simulink model "Simulink_Modell"  (R2020b)
settings: Solver=VariableStepAuto  StartTime=0.0  StopTime=1  MaxStep=0.000125  RelTol=1e-4  AbsTol=0.0000001
libraries: pid_lib x2
settings Model: Creator=Mei  LastModifiedBy=16007

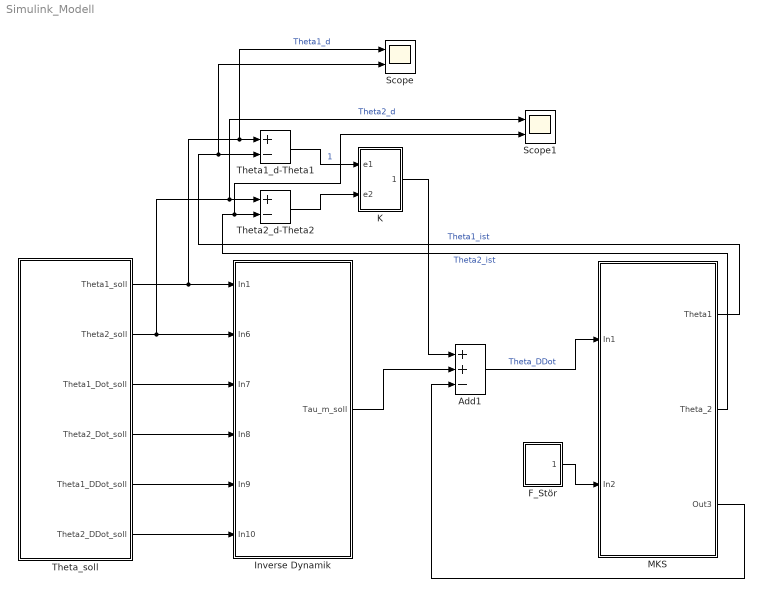
== system Simulink_Modell ==
  Add1 : Sum  Inputs=++-
  F_Stör : Subsystem
  Inverse Dynamik : Subsystem
  K : Subsystem
  MKS : Subsystem
  Scope : Scope  NumInputPorts=2
  Scope1 : Scope  NumInputPorts=2
  Theta1_d-Theta1 : Sum  Inputs=+-
  Theta2_d-Theta2 : Sum  Inputs=+-
  Theta_soll : Subsystem
  wires:
  Theta_soll/1(Theta1_soll) -> Scope/1, Theta1_d-Theta1/1, Inverse Dynamik/1(In1)  "Theta1_d"
  Theta_soll/2(Theta2_soll) -> Scope1/1, Theta2_d-Theta2/1, Inverse Dynamik/2(In6)  "Theta2_d"
  Theta_soll/3(Theta1_Dot_soll) -> Inverse Dynamik/3(In7)
  Theta_soll/4(Theta2_Dot_soll) -> Inverse Dynamik/4(In8)
  Theta_soll/5(Theta1_DDot_soll) -> Inverse Dynamik/5(In9)
  Theta_soll/6(Theta2_DDot_soll) -> Inverse Dynamik/6(In10)
  Add1/1 -> MKS/1(In1)  "Theta_DDot"
  F_Stör/1(1) -> MKS/2(In2)
  MKS/1(Theta1) -> Scope/2, Theta1_d-Theta1/2  "Theta1_ist"
  MKS/2(Theta_2) -> Scope1/2, Theta2_d-Theta2/2  "Theta2_ist"
  Theta1_d-Theta1/1 -> K/1(e1)  "1"
  Theta2_d-Theta2/1 -> K/2(e2)
  K/1(Out1) -> Add1/1
  Inverse Dynamik/1(Tau_m_soll) -> Add1/2
  MKS/3(Out3) -> Add1/3

== system Simulink_Modell/F_Stör ==
  Constant8 : Constant
  MATLAB Function : MATLAB Function  TreatAsAtomicUnit=on
  1 : Outport
  wires:
  Constant8/1 -> MATLAB Function/1(u)
  MATLAB Function/1(Fstoer) -> 1/1

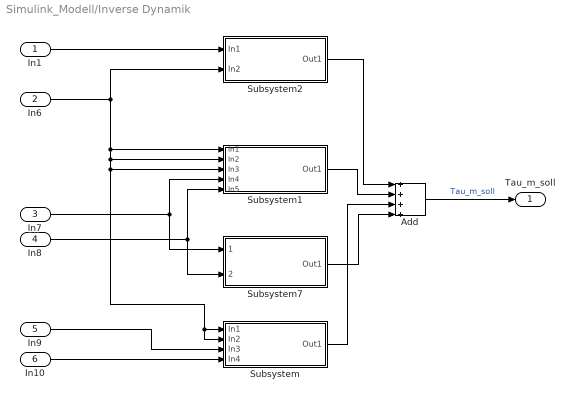
== system Simulink_Modell/Inverse Dynamik ==
  In1 : Inport
  In6 : Inport  Port=2
  In7 : Inport  Port=3
  In8 : Inport  Port=4
  In9 : Inport  Port=5
  In10 : Inport  Port=6
  Add : Sum  Inputs=++++
  Subsystem : Subsystem
  Subsystem1 : Subsystem
  Subsystem2 : Subsystem
  Subsystem7 : Subsystem
  Tau_m_soll : Outport
  wires:
  In7/1 -> Subsystem1/4(In4), Subsystem7/1(1)
  In8/1 -> Subsystem1/5(In5), Subsystem7/2(2)
  Add/1 -> Tau_m_soll/1  "Tau_m_soll"
  Subsystem/1(Out1) -> Add/3
  Subsystem1/1(Out1) -> Add/2
  Subsystem2/1(Out1) -> Add/1
  In6/1 -> Subsystem/2(In2), Subsystem/1(In1), Subsystem1/3(In3), Subsystem1/2(In2), Subsystem1/1(In1), Subsystem2/2(In2)
  Subsystem7/1(Out1) -> Add/4
  In1/1 -> Subsystem2/1(In1)
  In10/1 -> Subsystem/4(In4)
  In9/1 -> Subsystem/3(In3)

== system Simulink_Modell/K ==
  e1 : Inport
  e2 : Inport  Port=2
  Mux : Mux  Inputs=2
  PID1 : pid_lib/PID Controller  Controller=PID  Form=Parallel  TimeDomain=Discrete-time  UseExternalTs=off  SampleTime=-1  IntegratorMethod=Forward Euler  FilterMethod=Forward Euler  ControllerParametersSource=internal  P=300  I=10  D=10  UseFilter=on  N=100  TunerSelectOption=Transfer Function Based (PID Tuner App)  InitialConditionSource=internal  InitialConditionForIntegrator=0  InitialConditionForFilter=0  DifferentiatorICPrevScaledInput=0  ExternalReset=none  TrackingMode=off  Kt=1  LimitOutput=off  SatLimitsSource=internal  UpperSaturationLimit=inf  LowerSaturationLimit=-inf  LinearizeAsGain=on  AntiWindupMode=none  Kb=1  POutMin=[]  POutMax=[]  IOutMin=[]  IOutMax=[]  DOutMin=[]  DOutMax=[]  NOutMin=[]  NOutMax=[]  SumOutMin=[]  SumOutMax=[]  SaturationOutMin=[]  SaturationOutMax=[]  PParamMin=[]  PParamMax=[]  IParamMin=[]  IParamMax=[]  DParamMin=[]  DParamMax=[]  NParamMin=[]  NParamMax=[]  KbParamMin=[]  KbParamMax=[]  KtParamMin=[]  KtParamMax=[]  KbOutMin=[]  KbOutMax=[]  KtOutMin=[]  KtOutMax=[]  IntegratorOutMin=[]  IntegratorOutMax=[]  FilterOutMin=[]  FilterOutMax=[]  SumI1OutMin=[]  SumI1OutMax=[]  SumI2OutMin=[]  SumI2OutMax=[]  SumI3OutMin=[]  SumI3OutMax=[]  SumI4OutMin=[]  SumI4OutMax=[]  SumDOutMin=[]  SumDOutMax=[]  DifferentiatorOutMin=[]  DifferentiatorOutMax=[]  FilterDiffOutCoefMin=[]  FilterDiffOutCoefMax=[]  ReciprocalOutMin=[]  ReciprocalOutMax=[]  SumDenOutMin=[]  SumDenOutMax=[]  SumNumOutMin=[]  SumNumOutMax=[]  DivideOutMin=[]  DivideOutMax=[]  UdiffTsProdOutMin=[]  UdiffTsProdOutMax=[]  NTsProdOutMin=[]  NTsProdOutMax=[]  UintegralTsProdOutMin=[]  UintegralTsProdOutMax=[]  UngainTsProdOutMin=[]  UngainTsProdOutMax=[]  IntegratorContinuousStateAttributes=''  IntegratorStateMustResolveToSignalObject=off  IntegratorRTWStateStorageClass=Auto  FilterContinuousStateAttributes=''  FilterStateMustResolveToSignalObject=off  FilterRTWStateStorageClass=Auto  ParallelPVariant=InternalParameters  IdealPVariant=Disabled  IVariant=InternalParameters  DVariant=InternalParameters  IntegratorVariant=Discrete  SatVariant=Disabled  AWVariant=Passthrough  PCopyVariant=Disabled  TRVariant=Disabled  FdbkBlocksVariant=Forward  IdealPFdbkVariant=Disabled  SatFdbkVariant=Disabled  DerivativeFilterVariant=ForwardEulerFilter  NVariant=InternalParameters  NCopyVariant=Disabled  FilterICVariant=InternalICsFilter  IntegratorICVariant=InternalICs  ExternalResetVariant=Disabled  TRSumVariant=Passthrough  SumFdbkVariant=Disabled  SumVariant=Sum_PID  TsampFilterVariant=InternalTs  TsampNgainVariant=Passthrough  TsampIntegralVariant=Passthrough  ExternalSaturationOutDataTypeStr=Inherit: Same as second input
  PID2 : pid_lib/PID Controller  Controller=PID  Form=Parallel  TimeDomain=Discrete-time  UseExternalTs=off  SampleTime=-1  IntegratorMethod=Forward Euler  FilterMethod=Forward Euler  ControllerParametersSource=internal  P=1500  I=100  D=10  UseFilter=on  N=100  TunerSelectOption=Transfer Function Based (PID Tuner App)  InitialConditionSource=internal  InitialConditionForIntegrator=0  InitialConditionForFilter=0  DifferentiatorICPrevScaledInput=0  ExternalReset=none  TrackingMode=off  Kt=1  LimitOutput=off  SatLimitsSource=internal  UpperSaturationLimit=inf  LowerSaturationLimit=-inf  LinearizeAsGain=on  AntiWindupMode=none  Kb=1  POutMin=[]  POutMax=[]  IOutMin=[]  IOutMax=[]  DOutMin=[]  DOutMax=[]  NOutMin=[]  NOutMax=[]  SumOutMin=[]  SumOutMax=[]  SaturationOutMin=[]  SaturationOutMax=[]  PParamMin=[]  PParamMax=[]  IParamMin=[]  IParamMax=[]  DParamMin=[]  DParamMax=[]  NParamMin=[]  NParamMax=[]  KbParamMin=[]  KbParamMax=[]  KtParamMin=[]  KtParamMax=[]  KbOutMin=[]  KbOutMax=[]  KtOutMin=[]  KtOutMax=[]  IntegratorOutMin=[]  IntegratorOutMax=[]  FilterOutMin=[]  FilterOutMax=[]  SumI1OutMin=[]  SumI1OutMax=[]  SumI2OutMin=[]  SumI2OutMax=[]  SumI3OutMin=[]  SumI3OutMax=[]  SumI4OutMin=[]  SumI4OutMax=[]  SumDOutMin=[]  SumDOutMax=[]  DifferentiatorOutMin=[]  DifferentiatorOutMax=[]  FilterDiffOutCoefMin=[]  FilterDiffOutCoefMax=[]  ReciprocalOutMin=[]  ReciprocalOutMax=[]  SumDenOutMin=[]  SumDenOutMax=[]  SumNumOutMin=[]  SumNumOutMax=[]  DivideOutMin=[]  DivideOutMax=[]  UdiffTsProdOutMin=[]  UdiffTsProdOutMax=[]  NTsProdOutMin=[]  NTsProdOutMax=[]  UintegralTsProdOutMin=[]  UintegralTsProdOutMax=[]  UngainTsProdOutMin=[]  UngainTsProdOutMax=[]  IntegratorContinuousStateAttributes=''  IntegratorStateMustResolveToSignalObject=off  IntegratorRTWStateStorageClass=Auto  FilterContinuousStateAttributes=''  FilterStateMustResolveToSignalObject=off  FilterRTWStateStorageClass=Auto  ParallelPVariant=InternalParameters  IdealPVariant=Disabled  IVariant=InternalParameters  DVariant=InternalParameters  IntegratorVariant=Discrete  SatVariant=Disabled  AWVariant=Passthrough  PCopyVariant=Disabled  TRVariant=Disabled  FdbkBlocksVariant=Forward  IdealPFdbkVariant=Disabled  SatFdbkVariant=Disabled  DerivativeFilterVariant=ForwardEulerFilter  NVariant=InternalParameters  NCopyVariant=Disabled  FilterICVariant=InternalICsFilter  IntegratorICVariant=InternalICs  ExternalResetVariant=Disabled  TRSumVariant=Passthrough  SumFdbkVariant=Disabled  SumVariant=Sum_PID  TsampFilterVariant=InternalTs  TsampNgainVariant=Passthrough  TsampIntegralVariant=Passthrough  ExternalSaturationOutDataTypeStr=Inherit: Same as second input
  Out1 : Outport
  wires:
  PID1/1 -> Mux/1
  e1/1 -> PID1/1
  PID2/1 -> Mux/2
  e2/1 -> PID2/1
  Mux/1 -> Out1/1

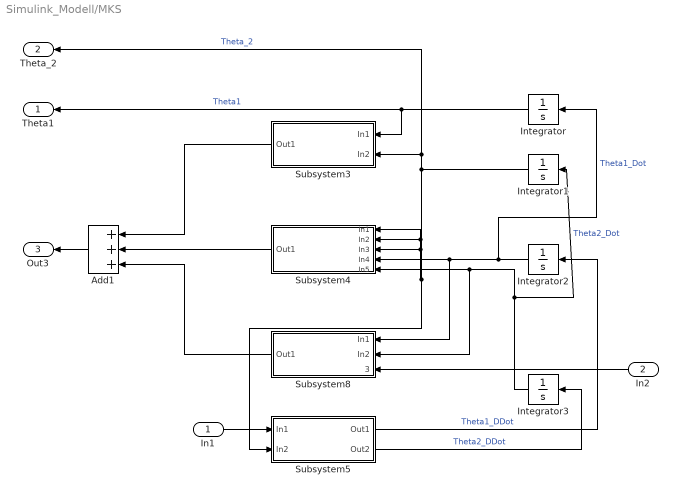
== system Simulink_Modell/MKS ==
  In1 : Inport
  In2 : Inport  Port=2
  Add1 : Sum  Inputs=+++
  Integrator{,1..3} (4 alike) : Integrator
  Subsystem3 : Subsystem
  Subsystem4 : Subsystem
  Subsystem5 : Subsystem
  Subsystem8 : Subsystem
  Theta1 : Outport
  Theta_2 : Outport  Port=2
  Out3 : Outport  Port=3
  wires:
  Integrator3/1 -> Integrator1/1, Subsystem4/5(In5), Subsystem8/2(In2)  "Theta2_Dot"
  Subsystem4/1(Out1) -> Add1/2
  Integrator2/1 -> Subsystem8/1(In1), Subsystem4/4(In4), Integrator/1  "Theta1_Dot"
  Subsystem5/2(Out2) -> Integrator3/1  "Theta2_DDot"
  Integrator1/1 -> Subsystem4/1(In1), Subsystem4/2(In2), Subsystem4/3(In3), Subsystem5/2(In2), Theta_2/1, Subsystem3/2(In2)  "Theta_2"
  Integrator/1 -> Theta1/1, Subsystem3/1(In1)  "Theta1"
  Subsystem5/1(Out1) -> Integrator2/1  "Theta1_DDot"
  In1/1 -> Subsystem5/1(In1)
  Subsystem3/1(Out1) -> Add1/1
  Subsystem8/1(Out1) -> Add1/3
  In2/1 -> Subsystem8/3(3)
  Add1/1 -> Out3/1

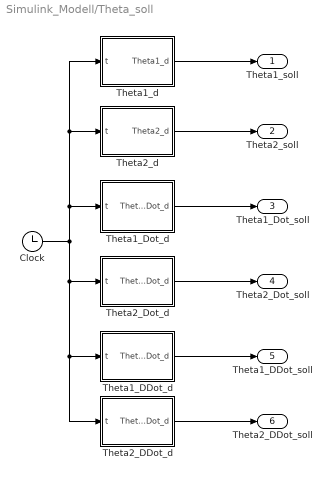
== system Simulink_Modell/Theta_soll ==
  Clock : Clock
  Theta1_DDot_d : MATLAB Function  TreatAsAtomicUnit=on
  Theta1_Dot_d : MATLAB Function  TreatAsAtomicUnit=on
  Theta1_d : MATLAB Function  TreatAsAtomicUnit=on
  Theta2_DDot_d : MATLAB Function  TreatAsAtomicUnit=on
  Theta2_Dot_d : MATLAB Function  TreatAsAtomicUnit=on
  Theta2_d : MATLAB Function  TreatAsAtomicUnit=on
  Theta1_soll : Outport
  Theta2_soll : Outport  Port=2
  Theta1_Dot_soll : Outport  Port=3
  Theta2_Dot_soll : Outport  Port=4
  Theta1_DDot_soll : Outport  Port=5
  Theta2_DDot_soll : Outport  Port=6
  wires:
  Theta1_Dot_d/1(Theta1_Dot_d) -> Theta1_Dot_soll/1
  Clock/1 -> Theta1_d/1(t), Theta2_d/1(t), Theta1_Dot_d/1(t), Theta2_DDot_d/1(t), Theta1_DDot_d/1(t), Theta2_Dot_d/1(t)
  Theta1_DDot_d/1(Theta1_DDot_d) -> Theta1_DDot_soll/1
  Theta1_d/1(Theta1_d) -> Theta1_soll/1
  Theta2_DDot_d/1(Theta2_DDot_d) -> Theta2_DDot_soll/1
  Theta2_Dot_d/1(Theta2_Dot_d) -> Theta2_Dot_soll/1
  Theta2_d/1(Theta2_d) -> Theta2_soll/1

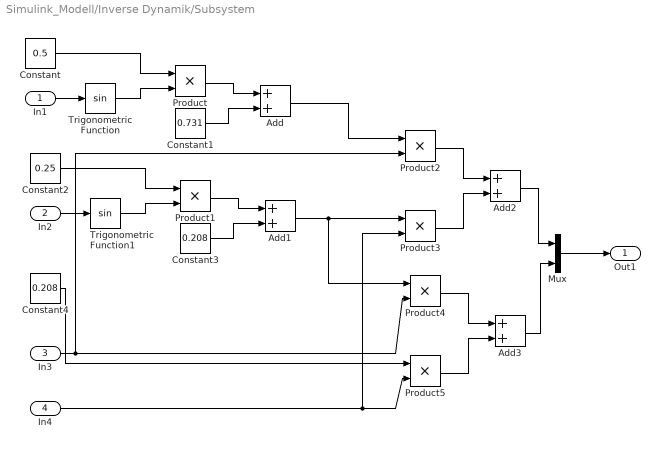
== system Simulink_Modell/Inverse Dynamik/Subsystem ==
  In1 : Inport
  In2 : Inport  Port=2
  In3 : Inport  Port=3
  In4 : Inport  Port=4
  Add{,1..3} (4 alike) : Sum
  Constant : Constant  Value=0.5
  Constant1 : Constant  Value=0.731
  Constant2 : Constant  Value=0.25
  Constant3 : Constant  Value=0.208
  Constant4 : Constant  Value=0.208
  Mux : Mux  Inputs=2
  Product{,1..5} (6 alike) : Product
  Trigonometric Function : Trigonometry
  Trigonometric Function1 : Trigonometry
  Out1 : Outport
  wires:
  Constant/1 -> Product/1
  Product/1 -> Add/1
  Constant1/1 -> Add/2
  In1/1 -> Trigonometric Function/1
  Trigonometric Function/1 -> Product/2
  Product1/1 -> Add1/1
  Constant3/1 -> Add1/2
  Constant2/1 -> Product1/1
  Trigonometric Function1/1 -> Product1/2
  In2/1 -> Trigonometric Function1/1
  In3/1 -> Product2/2, Product4/2
  Add/1 -> Product2/1
  Add1/1 -> Product4/1, Product3/1
  In4/1 -> Product3/2, Product5/2
  Product2/1 -> Add2/1
  Product3/1 -> Add2/2
  Product4/1 -> Add3/1
  Product5/1 -> Add3/2
  Constant4/1 -> Product5/1
  Add2/1 -> Mux/1
  Add3/1 -> Mux/2
  Mux/1 -> Out1/1

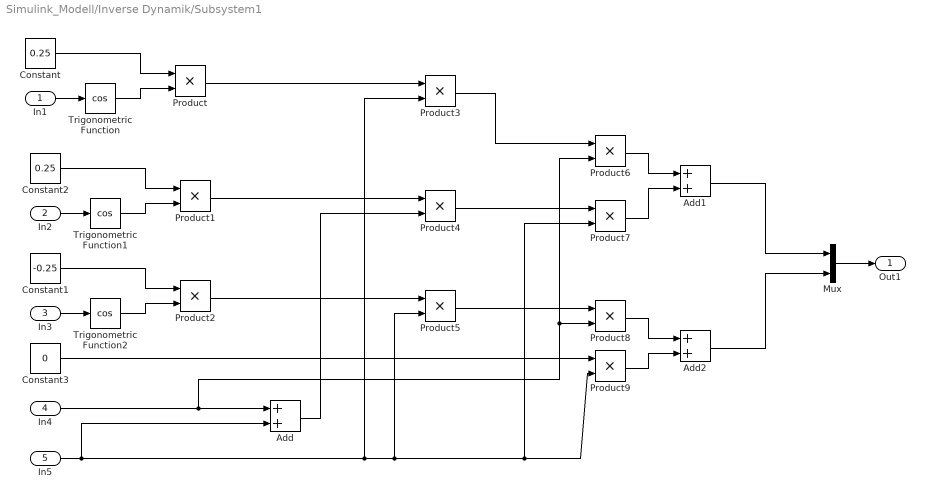
== system Simulink_Modell/Inverse Dynamik/Subsystem1 ==
  In1 : Inport
  In2 : Inport  Port=2
  In3 : Inport  Port=3
  In4 : Inport  Port=4
  In5 : Inport  Port=5
  Add : Sum
  Add1 : Sum
  Add2 : Sum
  Constant : Constant  Value=0.25
  Constant1 : Constant  Value=-0.25
  Constant2 : Constant  Value=0.25
  Constant3 : Constant  Value=0
  Mux : Mux  Inputs=2
  Product{,1..9} (10 alike) : Product
  Trigonometric Function : Trigonometry  Operator=cos
  Trigonometric Function1 : Trigonometry  Operator=cos
  Trigonometric Function2 : Trigonometry  Operator=cos
  Out1 : Outport
  wires:
  Constant/1 -> Product/1
  Trigonometric Function1/1 -> Product1/2
  Constant2/1 -> Product1/1
  In2/1 -> Trigonometric Function1/1
  Trigonometric Function/1 -> Product/2
  In1/1 -> Trigonometric Function/1
  In3/1 -> Trigonometric Function2/1
  Trigonometric Function2/1 -> Product2/2
  Constant1/1 -> Product2/1
  Product/1 -> Product3/1
  In5/1 -> Add/2, Product5/2, Product9/2, Product7/2, Product3/2
  Product1/1 -> Product4/1
  In4/1 -> Product6/2, Product8/2, Add/1
  Add/1 -> Product4/2
  Product2/1 -> Product5/1
  Product3/1 -> Product6/1
  Product4/1 -> Product7/1
  Product7/1 -> Add1/2
  Product6/1 -> Add1/1
  Product9/1 -> Add2/2
  Product8/1 -> Add2/1
  Product5/1 -> Product8/1
  Constant3/1 -> Product9/1
  Add2/1 -> Mux/2
  Add1/1 -> Mux/1
  Mux/1 -> Out1/1

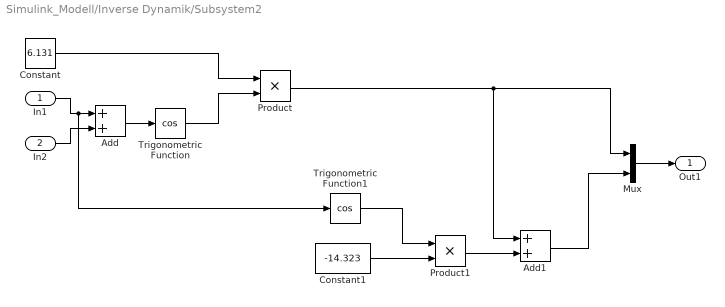
== system Simulink_Modell/Inverse Dynamik/Subsystem2 ==
  In1 : Inport
  In2 : Inport  Port=2
  Add : Sum
  Add1 : Sum
  Constant : Constant  Value=6.131
  Constant1 : Constant  Value=-14.323
  Mux : Mux  Inputs=2
  Product : Product
  Product1 : Product
  Trigonometric Function : Trigonometry  Operator=cos
  Trigonometric Function1 : Trigonometry  Operator=cos
  Out1 : Outport
  wires:
  Trigonometric Function/1 -> Product/2
  Constant/1 -> Product/1
  In1/1 -> Trigonometric Function1/1, Add/1
  In2/1 -> Add/2
  Add/1 -> Trigonometric Function/1
  Trigonometric Function1/1 -> Product1/1
  Constant1/1 -> Product1/2
  Product1/1 -> Add1/2
  Product/1 -> Mux/1, Add1/1
  Add1/1 -> Mux/2
  Mux/1 -> Out1/1

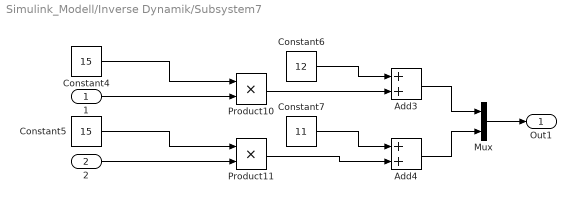
== system Simulink_Modell/Inverse Dynamik/Subsystem7 ==
  1 : Inport
  2 : Inport  Port=2
  Add3 : Sum
  Add4 : Sum
  Constant4 : Constant  Value=15
  Constant5 : Constant  Value=15
  Constant6 : Constant  Value=12
  Constant7 : Constant  Value=11
  Mux : Mux  Inputs=2
  Product10 : Product
  Product11 : Product
  Out1 : Outport
  wires:
  Constant6/1 -> Add3/1
  Product10/1 -> Add3/2
  Add3/1 -> Mux/1
  Constant7/1 -> Add4/1
  Product11/1 -> Add4/2
  Constant4/1 -> Product10/1
  2/1 -> Product11/2
  Constant5/1 -> Product11/1
  1/1 -> Product10/2
  Add4/1 -> Mux/2
  Mux/1 -> Out1/1

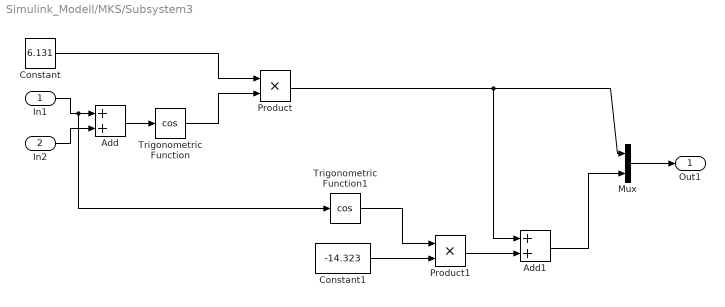
== system Simulink_Modell/MKS/Subsystem3 ==
  In1 : Inport
  In2 : Inport  Port=2
  Add : Sum
  Add1 : Sum
  Constant : Constant  Value=6.131
  Constant1 : Constant  Value=-14.323
  Mux : Mux  Inputs=2
  Product : Product
  Product1 : Product
  Trigonometric Function : Trigonometry  Operator=cos
  Trigonometric Function1 : Trigonometry  Operator=cos
  Out1 : Outport
  wires:
  Trigonometric Function/1 -> Product/2
  Constant/1 -> Product/1
  In1/1 -> Trigonometric Function1/1, Add/1
  In2/1 -> Add/2
  Add/1 -> Trigonometric Function/1
  Trigonometric Function1/1 -> Product1/1
  Constant1/1 -> Product1/2
  Product1/1 -> Add1/2
  Product/1 -> Mux/1, Add1/1
  Add1/1 -> Mux/2
  Mux/1 -> Out1/1

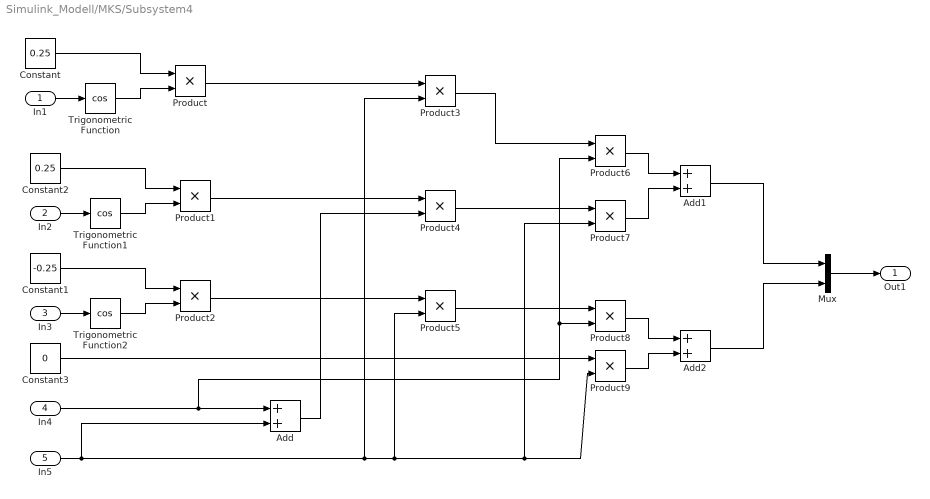
== system Simulink_Modell/MKS/Subsystem4 ==
  In1 : Inport
  In2 : Inport  Port=2
  In3 : Inport  Port=3
  In4 : Inport  Port=4
  In5 : Inport  Port=5
  Add : Sum
  Add1 : Sum
  Add2 : Sum
  Constant : Constant  Value=0.25
  Constant1 : Constant  Value=-0.25
  Constant2 : Constant  Value=0.25
  Constant3 : Constant  Value=0
  Mux : Mux  Inputs=2
  Product{,1..9} (10 alike) : Product
  Trigonometric Function : Trigonometry  Operator=cos
  Trigonometric Function1 : Trigonometry  Operator=cos
  Trigonometric Function2 : Trigonometry  Operator=cos
  Out1 : Outport
  wires:
  Constant/1 -> Product/1
  Trigonometric Function1/1 -> Product1/2
  Constant2/1 -> Product1/1
  In2/1 -> Trigonometric Function1/1
  Trigonometric Function/1 -> Product/2
  In1/1 -> Trigonometric Function/1
  In3/1 -> Trigonometric Function2/1
  Trigonometric Function2/1 -> Product2/2
  Constant1/1 -> Product2/1
  Product/1 -> Product3/1
  In5/1 -> Add/2, Product5/2, Product9/2, Product7/2, Product3/2
  Product1/1 -> Product4/1
  In4/1 -> Product6/2, Product8/2, Add/1
  Add/1 -> Product4/2
  Product2/1 -> Product5/1
  Product3/1 -> Product6/1
  Product4/1 -> Product7/1
  Product7/1 -> Add1/2
  Product6/1 -> Add1/1
  Product9/1 -> Add2/2
  Product8/1 -> Add2/1
  Product5/1 -> Product8/1
  Constant3/1 -> Product9/1
  Add2/1 -> Mux/2
  Add1/1 -> Mux/1
  Mux/1 -> Out1/1

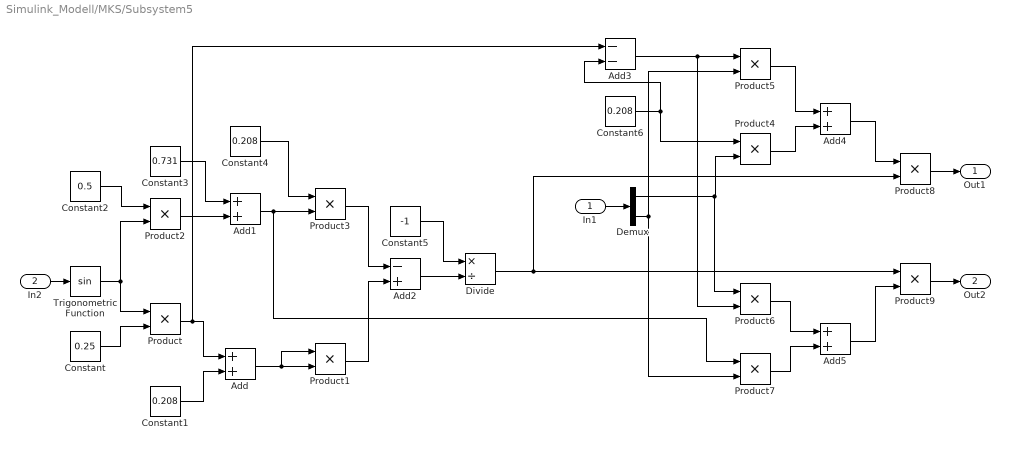
== system Simulink_Modell/MKS/Subsystem5 ==
  In1 : Inport
  In2 : Inport  Port=2
  Add{,1,4..5} (4 alike) : Sum
  Add2 : Sum  Inputs=-+
  Add3 : Sum  Inputs=--
  Constant : Constant  Value=0.25
  Constant1 : Constant  Value=0.208
  Constant2 : Constant  Value=0.5
  Constant3 : Constant  Value=0.731
  Constant4 : Constant  Value=0.208
  Constant5 : Constant  Value=-1
  Constant6 : Constant  Value=0.208
  Demux : Demux  Outputs=2
  Divide : Product  Inputs=*/
  Product{,1..9} (10 alike) : Product
  Trigonometric Function : Trigonometry
  Out1 : Outport
  Out2 : Outport  Port=2
  wires:
  In1/1 -> Demux/1
  In2/1 -> Trigonometric Function/1
  Trigonometric Function/1 -> Product2/2, Product/1
  Constant/1 -> Product/2
  Constant1/1 -> Add/2
  Product/1 -> Add3/1, Add/1
  Add/1 -> Product1/1, Product1/2
  Constant2/1 -> Product2/1
  Product2/1 -> Add1/2
  Constant3/1 -> Add1/1
  Add1/1 -> Product7/1, Product3/2
  Constant4/1 -> Product3/1
  Product1/1 -> Add2/2
  Product3/1 -> Add2/1
  Add2/1 -> Divide/2
  Constant5/1 -> Divide/1
  Constant6/1 -> Add3/2, Product4/1
  Demux/1 -> Product6/1, Product4/2
  Add3/1 -> Product5/1, Product6/2
  Demux/2 -> Product7/2, Product5/2
  Product5/1 -> Add4/1
  Product4/1 -> Add4/2
  Product6/1 -> Add5/1
  Product7/1 -> Add5/2
  Divide/1 -> Product9/1, Product8/2
  Add4/1 -> Product8/1
  Product8/1 -> Out1/1
  Add5/1 -> Product9/2
  Product9/1 -> Out2/1

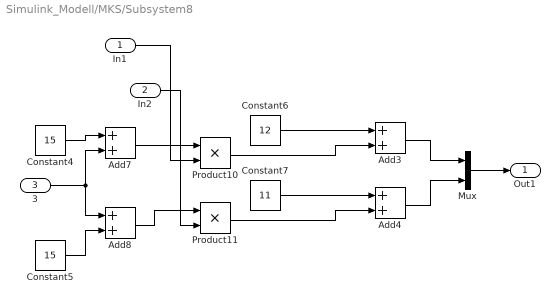
== system Simulink_Modell/MKS/Subsystem8 ==
  In1 : Inport
  In2 : Inport  Port=2
  3 : Inport  Port=3
  Add{3..4,7..8} (4 alike) : Sum
  Constant4 : Constant  Value=15
  Constant5 : Constant  Value=15
  Constant6 : Constant  Value=12
  Constant7 : Constant  Value=11
  Mux : Mux  Inputs=2
  Product10 : Product
  Product11 : Product
  Out1 : Outport
  wires:
  Constant5/1 -> Add8/2
  3/1 -> Add8/1, Add7/2
  Add8/1 -> Product11/1
  Product10/1 -> Add3/2
  Constant7/1 -> Add4/1
  Constant6/1 -> Add3/1
  Product11/1 -> Add4/2
  Constant4/1 -> Add7/1
  Add7/1 -> Product10/1
  Add4/1 -> Mux/2
  In2/1 -> Product11/2
  In1/1 -> Product10/2
  Add3/1 -> Mux/1
  Mux/1 -> Out1/1

== matlab function Simulink_Modell/Theta_soll/Theta1_d ==
  data: t input; Theta1_d output
function Theta1_d = fcn(t)
Theta1_d = -43.5*t.^2+29*t.^3;

== matlab function Simulink_Modell/Theta_soll/Theta1_Dot_d ==
  data: t input; Theta1_Dot_d output
function Theta1_Dot_d = fcn(t)
Theta1_Dot_d = -87*t+87*t^2;

== matlab function Simulink_Modell/Theta_soll/Theta2_Dot_d ==
  data: t input; Theta2_Dot_d output
function Theta2_Dot_d = fcn(t)
Theta2_Dot_d = 96*t-96*t^2;

== matlab function Simulink_Modell/Theta_soll/Theta1_DDot_d ==
  data: t input; Theta1_DDot_d output
function Theta1_DDot_d = fcn(t)
Theta1_DDot_d = -87+174*t;

== matlab function Simulink_Modell/Theta_soll/Theta2_DDot_d ==
  data: t input; Theta2_DDot_d output
function Theta2_DDot_d = fcn(t)
Theta2_DDot_d = 96-192*t;

== matlab function Simulink_Modell/F_Stör/MATLAB Function ==
  data: u input; Fstoer output
function Fstoer = fcn(u)
u=1;
Fstoer = -0.5 + 0.5*rand(u);

== matlab function Simulink_Modell/Theta_soll/Theta2_d ==
  data: t input; Theta2_d output
function Theta2_d = fcn(t)
Theta2_d = 48*t.^2 - 32*t.^3;
